simulink model "elecmechsim_og"  (R2025a)
settings: Solver=FixedStepAuto  StartTime=0.0  StopTime=100  FixedStep=0.001  RelTol=1e-3
undefined symbols (not defined in the file or in its folder): DiscIntNeverNeededParam
libraries: ee_lib x2, aerolibasang x1, sdl_lib x1, mpclib x1, simulink x1
settings Model: Creator=Fishyman  LastModifiedBy=crice

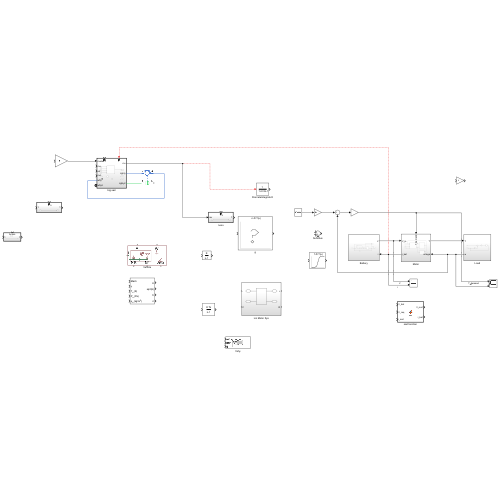
[thumbnail: Simulink's stored preview of the top-level diagram]
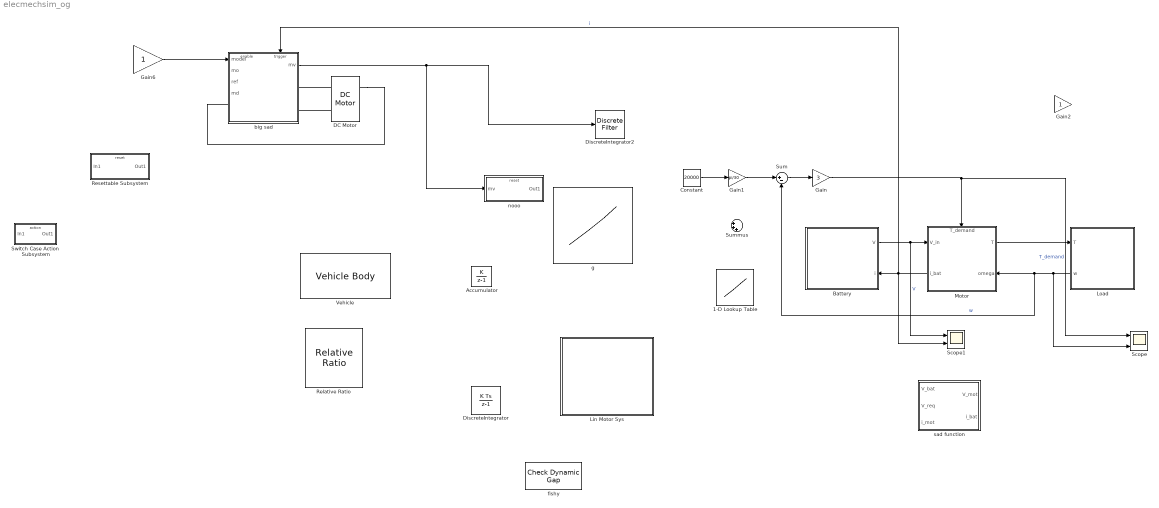
== system elecmechsim_og ==
  1-D Lookup Table : Lookup_n-D  NumberOfTableDimensions=1  BreakpointsForDimension1=[-5:5]  Table=tanh([-5:5])  InternalRulePriority=Speed  RndMeth=Simplest
  Accumulator : DiscreteIntegrator  IntegratorMethod=Accumulation: Forward Euler  SampleTime=-1  ICPrevOutput=DiscIntNeverNeededParam  ICPrevScaledInput=DiscIntNeverNeededParam
  Battery : Subsystem
      settings: PortSchema="{\"entries\":[{\"content\":{\"sides\":[{\"content\":{},\"type\":\"ConnectorPlacement.EquallySpacedRectSide\",\"uuid\":\"90dd6bea-f724-4f0e-b388-4faa47577b06\"},{\"content\":{\"connectorIds\":[\"Out1\",\"In1\"],\"side\":\"RIGHT\"},\"type\":\"ConnectorPlacement.EquallySpacedRectSide\",\"uuid\":\"c3b6cbe3-b84f-419e-9715-7957d7ea1c1e\"},{\"content\":{\"side\":\"TOP\"},\"type\":\"ConnectorPlacement.EquallySpacedRectSide\",\"uuid\":\"193a9e4d-398d-403b-bf54-6d04e8a510a2\"}]},\"type\":\"ConnectorPlacement.EquallySpacedConnector\",\"uuid\":\"ee056e4f-358f-4828-90d3-6930ea0d5628\"}],\"packageUris\":[\"http://schema.mathworks.com/mf0/Connector/R2020b\"],\"version\":\"1.0\"}"
  Constant : Constant  Value=20000
  DC Motor : ee_lib/Electromechanical/Brushed Motors/DC Motor  field_option=ee.enum.field_option.pm  Rf=100 Ohm  Lf=1 H  Laf=0.15 H  If0=0 A  parameterization=ee.enum.dcparam_option.circuit_param  Ra=3.9 Ohm  La=12e-6 H  emf_or_torque=ee.enum.emf_or_torque.kv  Kv=0.072e-3 V/rpm  Ki=6.876e-4 N*m/A  T_stall=0.24e-3 N*m  w_max=19100 rpm  w_rated=15000 rpm  P_rated=0.08 W  V_rated=1.5 V  lam_param=ee.enum.lam_param.damping  i_noload=0 A  V_i_noload=1.5 V  J=0.01 cm^2*g  lam=0 N*m*s/rad  speed0=0 rpm  alpha=3.93e-3 1/K  Tmeas=25 degC  thermal_mass=100 J/K  initial_temperature=25 degC
  DiscreteIntegrator : DiscreteIntegrator  ICPrevOutput=DiscIntNeverNeededParam  ICPrevScaledInput=DiscIntNeverNeededParam
  DiscreteIntegrator2 : DiscreteFilter
  Gain : Gain  Gain=3
  Gain1 : Gain  Gain=pi/30
  Gain2 : Gain
  Gain6 : Gain
  Lin Motor Sys : Subsystem
  Load : Subsystem
      settings: PortSchema="{\"entries\":[{\"content\":{\"sides\":[{\"content\":{\"connectorIds\":[\"In1\",\"Out1\"]},\"type\":\"ConnectorPlacement.EquallySpacedRectSide\",\"uuid\":\"90dd6bea-f724-4f0e-b388-4faa47577b06\"},{\"content\":{\"side\":\"RIGHT\"},\"type\":\"ConnectorPlacement.EquallySpacedRectSide\",\"uuid\":\"c3b6cbe3-b84f-419e-9715-7957d7ea1c1e\"},{\"content\":{\"side\":\"TOP\"},\"type\":\"ConnectorPlacement.EquallySpacedRectSide\",\"uuid\":\"193a9e4d-398d-403b-bf54-6d04e8a510a2\"}]},\"type\":\"ConnectorPlacement.EquallySpacedConnector\",\"uuid\":\"ee056e4f-358f-4828-90d3-6930ea0d5628\"}],\"packageUris\":[\"http://schema.mathworks.com/mf0/Connector/R2020b\"],\"version\":\"1.0\"}"
  Motor : Subsystem
      settings: PortSchema="{\"entries\":[{\"content\":{\"sides\":[{\"content\":{\"connectorIds\":[\"In1\",\"Out2\"]},\"type\":\"ConnectorPlacement.EquallySpacedRectSide\",\"uuid\":\"59bece3f-90cf-47e3-b7f7-45472b4ed29b\"},{\"content\":{\"connectorIds\":[\"Out1\",\"In3\"],\"side\":\"RIGHT\"},\"type\":\"ConnectorPlacement.EquallySpacedRectSide\",\"uuid\":\"a8762b20-55df-48c6-9a38-100f62965a72\"},{\"content\":{\"connectorIds\":[\"In2\"],\"side\":\"TOP\"},\"type\":\"ConnectorPlacement.EquallySpacedRectSide\",\"uuid\":\"f2b0052a-0f93-449a-a72f-4be1aa749add\"}]},\"type\":\"ConnectorPlacement.EquallySpacedConnector\",\"uuid\":\"3b29a972-b8e8-42da-9561-e1105daf668b\"}],\"packageUris\":[\"http://schema.mathworks.com/mf0/Connector/R2020b\"],\"version\":\"1.0\"}"
  Relative Ratio : aerolibasang/Relative Ratio  units=Metric (MKS)  theta=on  sq_theta=on  delta=on  sigma=on
  Resettable Subsystem : Subsystem  TreatAsAtomicUnit=on
  Scope : Scope  NumInputPorts=3
      settings: ActiveDisplayYMinimum=5708.76635  ActiveDisplayYMaximum=6347.00964
  Scope1 : Scope  NumInputPorts=2
      settings: ActiveDisplayYMinimum=40.25471  ActiveDisplayYMaximum=42.74948
  Sum : Sum  Inputs=|+-
  Summus : Sum  Inputs=|+++
  Switch Case Action Subsystem : Subsystem  TreatAsAtomicUnit=on
  Vehicle : sdl_lib/Tires & Vehicles/Vehicle Body  mass=1200 kg  n_w=2  x_f=1.4 m  x_r=1.6 m  y_c=0.5 m  mass_var=false  g=9.81 m/s^2  liftoff_warning=false  area=3 m^2  Cd_var=false  Cd=0.4  rho=1.18 kg/m^3  model_pitch=false  inertia=4000 kg*m^2  suspension_model=sdl.enum.linearTLU.linear  k_f=1e4 N/m  b_f=1e4 N*s/m  k_r=1e4 N/m  b_r=1e4 N*s/m  k_f_TLU=[-2000, -1000, 0, 1000, 2000] N  x_f_TLU=[-.4, -.2, 0, .2, .4] m  b_f_TLU=[-200, -100, 0, 100, 200] N  v_f_TLU=[-4, -2, 0, 2, 4] m/s  k_r_TLU=[-2000, -1000, 0, 1000, 2000] N  x_r_TLU=[-.4, -.2, 0, .2, .4] m  b_r_TLU=[-200, -100, 0, 100, 200] N  v_r_TLU=[-4, -2, 0, 2, 4] m/s  interp_method=simscape.enum.interpolation.linear  extrap_method=simscape.enum.extrapolation.linear  model_hardstop=false  upper_bound_f=.25 m  lower_bound_f=-.25 m  stop_k_f=1e6 N/m  stop_b_f=150 N*s/m  upper_bound_r=.25 m  lower_bound_r=-.25 m  stop_k_r=1e6 N/m  stop_b_r=150 N*s/m  initial_pitch=0 rad  initial_pitch_rate=0 rad/s  v_specify=off  v_priority=High  v=0 m/s  v_nominal_specify=off  v_nominal_value=1  v_nominal_unit=m/s
      settings: InternalSimscapePortConfiguration="{\"Bottom\":[{\"id\":\"NR\",\"label\":\"NR\",\"type\":\"output\"},{\"id\":\"NF\",\"label\":\"NF\",\"type\":\"output\"},{\"id\":\"beta\",\"label\":\"beta\",\"type\":\"input\"}],\"Left\":[{\"id\":\"H\",\"label\":\"H\",\"type\":\"foundation.mechanical.translational.translational\"}],\"Right\":[],\"Top\":[{\"id\":\"V\",\"label\":\"V\",\"type\":\"output\"},{\"id\":\"wind\",\"label\":\"W\",\"type\":\"input\"}]}"
  big sad : Subsystem
  fishy : simulink/Model Verification/Check  Dynamic Gap  Description=u < min || max < u  enabled=on  stopWhenAssertionFail=on  export=off  icon=graphic
  g : Lookup_n-D  NumberOfTableDimensions=1
  nooo : Subsystem  TreatAsAtomicUnit=on
  sad function : MATLAB Function  TreatAsAtomicUnit=on
  wires:
  Battery/1(V) -> Scope1/1, Motor/1(V_in)  "V"
  Motor/2(i_bat) -> big sad/Trigger, Scope1/2, Battery/1(i)  "i"
  Load/1(w) -> Scope/3, Sum/2, Motor/3(omega)  "w"
  Sum/1 -> Gain/1
  Constant/1 -> Gain1/1
  Gain/1 -> Scope/1, Motor/2(T_demand)  "T_demand"
  Gain1/1 -> Sum/1
  Motor/1(T) -> Load/1(T)
  Gain6/1 -> big sad/1(model)
  big sad/1(mv) -> nooo/1(mv), DiscreteIntegrator2/1
  connections:
  DC Motor/RConn1 -- big sad/RConn1
  DC Motor/LConn1 -- big sad/LConn1
  DC Motor/RConn2 -- big sad/RConn2

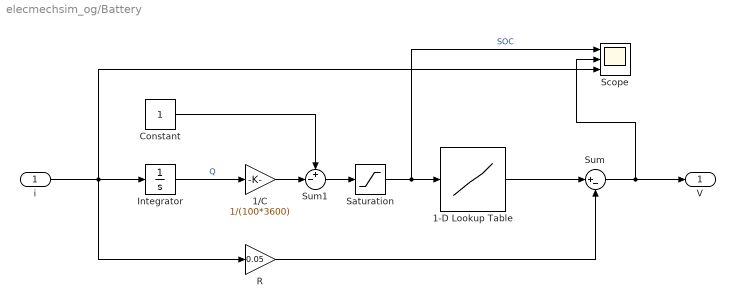
== system elecmechsim_og/Battery ==
  i : Inport
  1-D Lookup Table : Lookup_n-D  NumberOfTableDimensions=1  BreakpointsForDimension1=[0, 0.15, 0.2, 0.8, 0.95, 1]  Table=[22.5, 35, 37.5, 37.5, 40, 42.5]  InternalRulePriority=Speed  RndMeth=Simplest
  1/C : Gain  Gain=1/(100*3600)
  Constant : Constant
  Integrator : Integrator
  R : Gain  Gain=0.05
  Saturation : Saturate  UpperLimit=1  LowerLimit=0
  Scope : Scope  NumInputPorts=3
      settings: ActiveDisplayYMinimum=0.99078  ActiveDisplayYMaximum=1.00102  DataLoggingVariableName=ScopeData4
  Sum : Sum  Inputs=|+-
  Sum1 : Sum  Inputs=+-|
  V : Outport
  wires:
  Constant/1 -> Sum1/1
  i/1 -> R/1, Scope/3, Integrator/1
  1-D Lookup Table/1 -> Sum/1
  Integrator/1 -> 1/C/1  "Q"
  Saturation/1 -> Scope/1, 1-D Lookup Table/1  "SOC"
  Sum1/1 -> Saturation/1
  Sum/1 -> Scope/2, V/1
  1/C/1 -> Sum1/2
  R/1 -> Sum/2

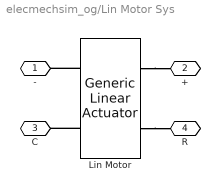
== system elecmechsim_og/Lin Motor Sys ==
  Lin Motor : ee_lib/Electromechanical/Mechatronic Actuators/Generic Linear Actuator  v_vec=[-15, -10, -5, 0, 5, 10, 15, 20, 25, 30] m/s  F_vec=[4, 3.5, 3, 2.5, 2, 1.5, 1, .5, 0, -.5] N  Vrated=12 V  eff=70  Pbase=2 W  pwm_or_av=ee.enum.pwm_or_av.pwm  v_eff=20 m/s  Mass=0.1 kg  lam=1e-5 N*s/m  i_specify=off  i_priority=None  i=0 A  i_nominal_specify=off  i_nominal_value=1  i_nominal_unit=A  f_specify=off  f_priority=None  f=0 N  f_nominal_specify=off  f_nominal_value=1  f_nominal_unit=N  velocity_specify=off  velocity_priority=None  velocity=0 m/s  velocity_nominal_specify=off  velocity_nominal_value=1  velocity_nominal_unit=m/s  alpha=3.93e-3 1/K  Tmeas=25 degC  thermal_mass=100 J/K  Q_specify=off  Q_priority=None  Q=0 W  Q_nominal_specify=off  Q_nominal_value=1  Q_nominal_unit=W  temperature_specify=off  temperature_priority=High  temperature=300 K  temperature_nominal_specify=off  temperature_nominal_value=1  temperature_nominal_unit=K
      settings: InternalSimscapePortConfiguration="{\"Bottom\":[],\"Left\":[{\"id\":\"p\",\"label\":\"+\",\"type\":\"foundation.electrical.electrical\"},{\"id\":\"R\",\"label\":\"R\",\"type\":\"foundation.mechanical.translational.translational\"}],\"Right\":[{\"id\":\"n\",\"label\":\"-\",\"type\":\"foundation.electrical.electrical\"},{\"id\":\"C\",\"label\":\"C\",\"type\":\"foundation.mechanical.translational.translational\"}],\"Top\":[]}"
  - : PMIOPort  Side=Right
  + : PMIOPort  Port=2  Side=Left
  C : PMIOPort  Port=3  Side=Right
  R : PMIOPort  Port=4  Side=Left
  connections:
  Lin Motor/RConn1 -- -/RConn1
  Lin Motor/LConn1 -- +/RConn1
  Lin Motor/LConn2 -- R/RConn1
  Lin Motor/RConn2 -- C/RConn1

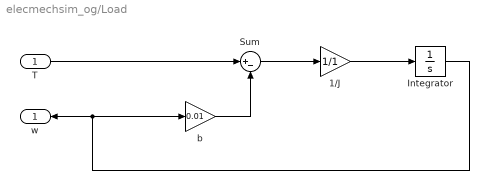
== system elecmechsim_og/Load ==
  T : Inport
  1/J : Gain  Gain=1/1
  Integrator : Integrator
  Sum : Sum  Inputs=|+-
  b : Gain  Gain=0.01
  w : Outport
  wires:
  1/J/1 -> Integrator/1
  Sum/1 -> 1/J/1
  Integrator/1 -> b/1, w/1
  T/1 -> Sum/1
  b/1 -> Sum/2

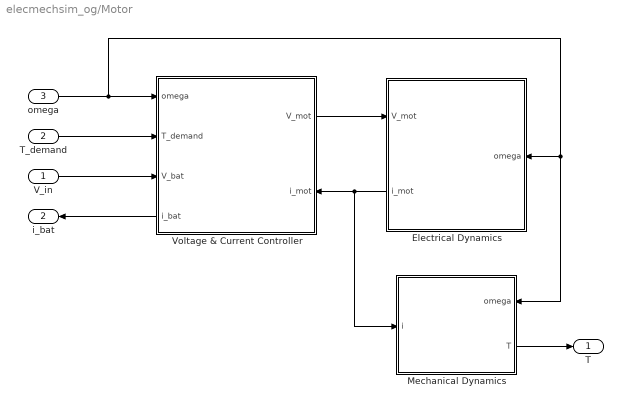
== system elecmechsim_og/Motor ==
  V_in : Inport
  T_demand : Inport  Port=2
  omega : Inport  Port=3
  Electrical Dynamics : Subsystem
      settings: PortSchema="{\"entries\":[{\"content\":{\"sides\":[{\"content\":{\"connectorIds\":[\"In1\",\"Out1\"]},\"type\":\"ConnectorPlacement.EquallySpacedRectSide\",\"uuid\":\"e446b3b9-b6cf-41bb-9ba1-a3aa4740c662\"},{\"content\":{\"connectorIds\":[\"In2\"],\"side\":\"RIGHT\"},\"type\":\"ConnectorPlacement.EquallySpacedRectSide\",\"uuid\":\"73556d2e-6dbd-43bd-8be5-c816eca01439\"},{\"content\":{\"side\":\"TOP\"},\"type\":\"ConnectorPlacement.EquallySpacedRectSide\",\"uuid\":\"80b3db30-baf9-488a-ad9e-05e46134b456\"},{\"content\":{\"side\":\"BOTTOM\"},\"type\":\"ConnectorPlacement.EquallySpacedRectSide\",\"uuid\":\"2369e07d-0029-49e3-9a6d-e102a23332b5\"}]},\"type\":\"ConnectorPlacement.EquallySpacedConnector\",\"uuid\":\"1c7cf443-8404-434d-b421-a5c7aaa92c5d\"}],\"packageUris\":[\"http://schema.mathworks.com/mf0/Connector/R2020b\"],\"version\":\"1.0\"}"
  Mechanical Dynamics : Subsystem
      settings: PortSchema="{\"entries\":[{\"content\":{\"sides\":[{\"content\":{\"connectorIds\":[\"In1\"]},\"type\":\"ConnectorPlacement.EquallySpacedRectSide\",\"uuid\":\"e446b3b9-b6cf-41bb-9ba1-a3aa4740c662\"},{\"content\":{\"connectorIds\":[\"In2\",\"Out1\"],\"side\":\"RIGHT\"},\"type\":\"ConnectorPlacement.EquallySpacedRectSide\",\"uuid\":\"73556d2e-6dbd-43bd-8be5-c816eca01439\"},{\"content\":{\"side\":\"TOP\"},\"type\":\"ConnectorPlacement.EquallySpacedRectSide\",\"uuid\":\"80b3db30-baf9-488a-ad9e-05e46134b456\"}]},\"type\":\"ConnectorPlacement.EquallySpacedConnector\",\"uuid\":\"1c7cf443-8404-434d-b421-a5c7aaa92c5d\"}],\"packageUris\":[\"http://schema.mathworks.com/mf0/Connector/R2020b\"],\"version\":\"1.0\"}"
  Voltage & Current Controller : Subsystem
      settings: PortSchema="{\"entries\":[{\"content\":{\"sides\":[{\"content\":{\"connectorIds\":[\"In1\",\"In2\",\"In3\",\"Out2\"]},\"type\":\"ConnectorPlacement.EquallySpacedRectSide\",\"uuid\":\"7386bc59-c7cf-4e24-a03c-2c63c88805fb\"},{\"content\":{\"connectorIds\":[\"Out1\",\"In4\"],\"side\":\"RIGHT\"},\"type\":\"ConnectorPlacement.EquallySpacedRectSide\",\"uuid\":\"9d9f903b-7c00-446f-883d-5e6a0c4fe953\"},{\"content\":{\"side\":\"TOP\"},\"type\":\"ConnectorPlacement.EquallySpacedRectSide\",\"uuid\":\"243b84c1-c409-4364-aedd-e89918ead118\"}]},\"type\":\"ConnectorPlacement.EquallySpacedConnector\",\"uuid\":\"f42fac57-5517-4d2b-831b-44217276121d\"}],\"packageUris\":[\"http://schema.mathworks.com/mf0/Connector/R2020b\"],\"version\":\"1.0\"}"
  T : Outport
  i_bat : Outport  Port=2
  wires:
  V_in/1 -> Voltage & Current Controller/3(V_bat)
  T_demand/1 -> Voltage & Current Controller/2(T_demand)
  Mechanical Dynamics/1(T) -> T/1
  Voltage & Current Controller/2(i_bat) -> i_bat/1
  Voltage & Current Controller/1(V_mot) -> Electrical Dynamics/1(V_mot)
  Electrical Dynamics/1(i_mot) -> Mechanical Dynamics/1(i), Voltage & Current Controller/4(i_mot)
  omega/1 -> Electrical Dynamics/2(omega), Mechanical Dynamics/2(omega), Voltage & Current Controller/1(omega)

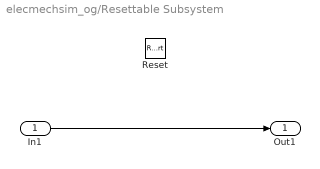
== system elecmechsim_og/Resettable Subsystem ==
  In1 : Inport
  Reset : ResetPort  DisableCoverage=on
  Out1 : Outport
  wires:
  In1/1 -> Out1/1

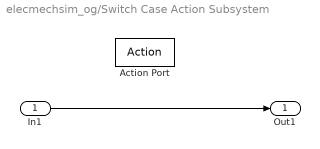
== system elecmechsim_og/Switch Case Action Subsystem ==
  In1 : Inport
  Action Port : ActionPort
  Out1 : Outport
  wires:
  In1/1 -> Out1/1

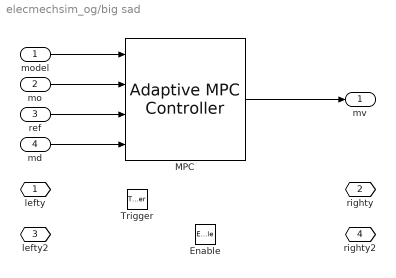
== system elecmechsim_og/big sad ==
  model : Inport
  mo : Inport  Port=2
  ref : Inport  Port=3
  md : Inport  Port=4
  Enable : EnablePort
  Trigger : TriggerPort  VariantControl=(inherit)  PortDimensions=1
  MPC : mpclib/Adaptive MPC Controller  SCDEnableBlockLinearizationSpecification=on  enable_value=0  updateMPCinCallerWorkspace=on  md_inport=on  mv_inport=off  uref_inport=off  return_cost=off  return_mvseq=off  return_qpstatus=off  return_xseq=off  return_state=off  return_ovseq=off  state_inport=off  isltv_plant=off  umin_inport=off  umax_inport=off  ymin_inport=off  ymax_inport=off  cc_inport=off  ywt_inport=off  uwt_inport=off  duwt_inport=off  rhoeps_inport=off  pm_inport=off  MaximumP=10  HorizonChoice=FixedHorizon  BlockDataType=double  SampleTimeInherited=off  switch_inport=off
  lefty : PMIOPort  Side=Left
  righty : PMIOPort  Port=2  Side=Right
  lefty2 : PMIOPort  Port=3  Side=Left
  righty2 : PMIOPort  Port=4  Side=Right
  mv : Outport
  wires:
  MPC/1 -> mv/1
  model/1 -> MPC/1
  mo/1 -> MPC/2
  ref/1 -> MPC/3
  md/1 -> MPC/4

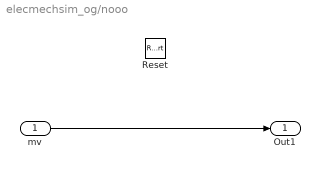
== system elecmechsim_og/nooo ==
  mv : Inport
  Reset : ResetPort  DisableCoverage=on
  Out1 : Outport
  wires:
  mv/1 -> Out1/1

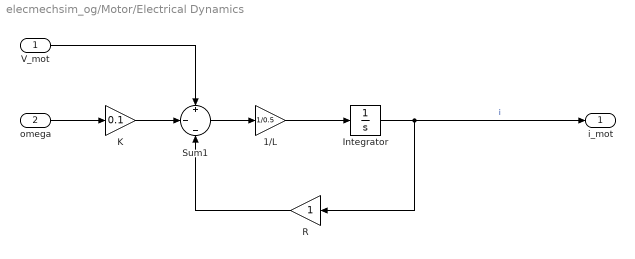
== system elecmechsim_og/Motor/Electrical Dynamics ==
  V_mot : Inport
  omega : Inport  Port=2
  1/L : Gain  Gain=1/0.5
  Integrator : Integrator
  K : Gain  Gain=0.1
  R : Gain
  Sum1 : Sum  Inputs=+|-|-
  i_mot : Outport
  wires:
  Integrator/1 -> R/1, i_mot/1  "i"
  Sum1/1 -> 1/L/1
  K/1 -> Sum1/2
  omega/1 -> K/1
  R/1 -> Sum1/3
  1/L/1 -> Integrator/1
  V_mot/1 -> Sum1/1

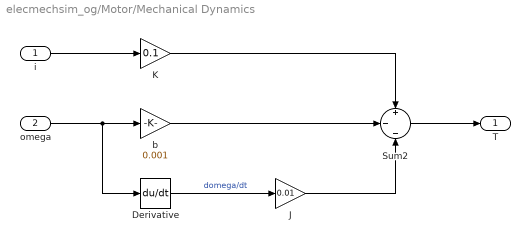
== system elecmechsim_og/Motor/Mechanical Dynamics ==
  i : Inport
  omega : Inport  Port=2
  Derivative : Derivative
  J : Gain  Gain=0.01
  K : Gain  Gain=0.1
  Sum2 : Sum  Inputs=+|-|-
  b : Gain  Gain=0.001
  T : Outport
  wires:
  Derivative/1 -> J/1  "domega/dt"
  b/1 -> Sum2/2
  K/1 -> Sum2/1
  omega/1 -> Derivative/1, b/1
  i/1 -> K/1
  J/1 -> Sum2/3
  Sum2/1 -> T/1

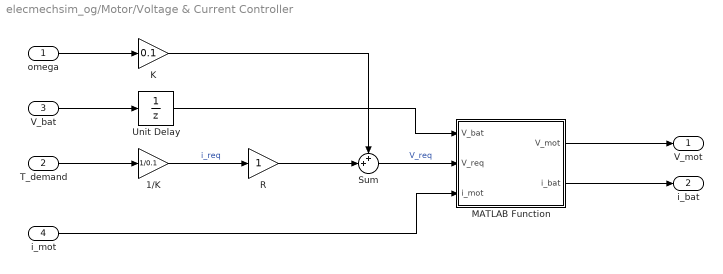
== system elecmechsim_og/Motor/Voltage & Current Controller ==
  omega : Inport
  T_demand : Inport  Port=2
  V_bat : Inport  Port=3
  i_mot : Inport  Port=4
  1/K : Gain  Gain=1/0.1
  K : Gain  Gain=0.1
  MATLAB Function : MATLAB Function  TreatAsAtomicUnit=on
  R : Gain
  Sum : Sum  Inputs=++|
  Unit Delay : UnitDelay  SampleTime=-1  HasFrameUpgradeWarning=on
  V_mot : Outport
  i_bat : Outport  Port=2
  wires:
  V_bat/1 -> Unit Delay/1
  R/1 -> Sum/2
  1/K/1 -> R/1  "i_req"
  K/1 -> Sum/1
  T_demand/1 -> 1/K/1
  omega/1 -> K/1
  Unit Delay/1 -> MATLAB Function/1(V_bat)
  Sum/1 -> MATLAB Function/2(V_req)  "V_req"
  i_mot/1 -> MATLAB Function/3(i_mot)
  MATLAB Function/1(V_mot) -> V_mot/1
  MATLAB Function/2(i_bat) -> i_bat/1

== matlab function elecmechsim_og/sad function ==
  data: V_bat input; V_req input; V_mot output; i_mot input; i_bat output
function [V_mot, i_bat]= fcn(V_bat, V_req, i_mot)

V_mot = min(max(-V_bat, V_req), V_bat);
if V_bat == 0
    i_bat = 0;
else 
    i_bat = (V_mot * i_mot) / V_bat;
end

== matlab function elecmechsim_og/Motor/Voltage & Current Controller/MATLAB Function ==
  data: V_bat input; V_req input; V_mot output; i_mot input; i_bat output
function [V_mot, i_bat]= fcn(V_bat, V_req, i_mot)

V_mot = min(max(-V_bat, V_req), V_bat);
if V_bat == 0
    i_bat = 0;
else 
    i_bat = (V_mot * i_mot) / V_bat;
end
